simulink model "Motor_Load"  (R2025b)
settings: Solver=VariableStepAuto  StartTime=0.0  StopTime=400  MaxStep=0.002  RelTol=1e-3
model workspace (MAT data in the model file):
  CS_area_of_vehicle = 0.871
  Drag_coefficient = 0.195
  acceleration = 2.5
  air_density = 1.225
  gear_ratio = 5
  gravity = 9.81
  rolling_resistance = 0.05
  vehicle_mass = 180
  wheel_radius = 0.25
undefined symbols (not defined in the file or in its folder): Gradient_data, PMSM_Graph
settings Model: Creator=User  LastModifiedBy=User

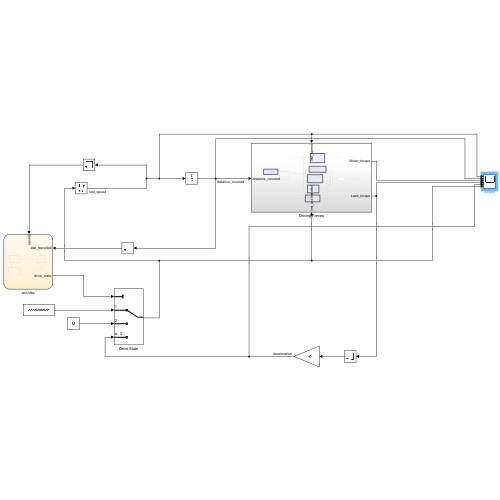
[thumbnail: Simulink's stored preview of the top-level diagram]
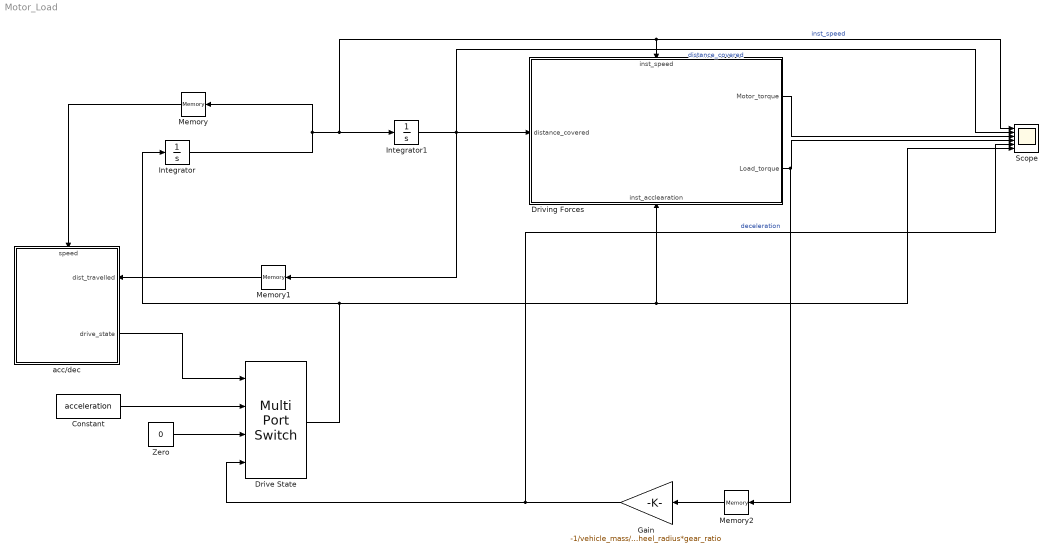
== system Motor_Load ==
  Constant : Constant  Value=acceleration
  Drive State : MultiPortSwitch  DataPortOrder=Specify indices  SaturateOnIntegerOverflow=off  InputSameDT=off
  Driving Forces : Subsystem
      settings: PortSchema="{\"entries\":[{\"content\":{\"sides\":[{\"content\":{\"connectorIds\":[\"In1\"]},\"type\":\"ConnectorPlacement.EquallySpacedRectSide\",\"uuid\":\"0ef3818d-e5de-4410-93cb-475bf6d7adfa\"},{\"content\":{\"connectorIds\":[\"Out1\",\"Out2\"],\"side\":\"RIGHT\"},\"type\":\"ConnectorPlacement.EquallySpacedRectSide\",\"uuid\":\"9d154a41-18f4-4f0c-ab8b-f09b7ff3397b\"},{\"content\":{\"connectorIds\":[\"In2\"],\"side\":\"TOP\"},\"type\":\"ConnectorPlacement.EquallySpacedRectSide\",\"uuid\":\"d46c2e69-b7e7-4a8c-bdbb-3c3b035d244f\"},{\"content\":{\"connectorIds\":[\"In3\"],\"side\":\"BOTTOM\"},\"type\":\"ConnectorPlacement.EquallySpacedRectSide\",\"uuid\":\"b2e27950-85a1-4e60-a0a3-1e85ddf78ec7\"}]},\"type\":\"ConnectorPlacement.EquallySpacedConnector\",\"uuid\":\"c1717862-f1cf-4e53-be39-73b9e4c32012\"}],\"packageUris\":[\"http://schema.mathworks.com/mf0/Connector/R2020b\"],\"version\":\"1.0\"}"
  Gain : Gain  Gain=-1/vehicle_mass/wheel_radius*gear_ratio
  Integrator : Integrator  InitialCondition=0.001  LimitOutput=on  UpperSaturationLimit=10  LowerSaturationLimit=-0.001
  Integrator1 : Integrator
  Memory : Memory
  Memory1 : Memory
  Memory2 : Memory
  Scope : Scope  NumInputPorts=6
      settings: ActiveDisplayYMinimum=-26.829853892938957  ActiveDisplayYMaximum=39.839891777673373
  Zero : Constant  Value=0  OutDataTypeStr=Inherit: Inherit via back propagation
  acc/dec : Stateflow chart  TreatAsAtomicUnit=on
      settings: PortSchema="{\"entries\":[{\"content\":{\"sides\":[{\"content\":{},\"type\":\"ConnectorPlacement.EquallySpacedRectSide\",\"uuid\":\"4b427815-5634-4ea7-8cfa-82438ecc852b\"},{\"content\":{\"connectorIds\":[\"In1\",\"Out1\"],\"side\":\"RIGHT\"},\"type\":\"ConnectorPlacement.EquallySpacedRectSide\",\"uuid\":\"a8ca7e8d-f0e3-4217-abff-5b21a522cee7\"},{\"content\":{\"connectorIds\":[\"In2\"],\"side\":\"TOP\"},\"type\":\"ConnectorPlacement.EquallySpacedRectSide\",\"uuid\":\"3ab37e47-b840-4f90-8038-0626af8ff66b\"}]},\"type\":\"ConnectorPlacement.EquallySpacedConnector\",\"uuid\":\"434126e8-21ff-4afc-bfcf-7bdbff78af77\"}],\"packageUris\":[\"http://schema.mathworks.com/mf0/Connector/R2020b\"],\"version\":\"1.0\"}"
  wires:
  Integrator/1 -> Memory/1, Integrator1/1, Scope/1, Driving Forces/2(inst_speed)  "inst_speed"
  Integrator1/1 -> Scope/2, Memory1/1, Driving Forces/1(distance_covered)  "distance_covered"
  Constant/1 -> Drive State/2
  acc/dec/1(drive_state) -> Drive State/1
  Gain/1 -> Scope/5, Drive State/4  "deceleration"
  Drive State/1 -> Driving Forces/3(inst_acclearation), Scope/6, Integrator/1
  Driving Forces/2(Load_torque) -> Memory2/1, Scope/4
  Driving Forces/1(Motor_torque) -> Scope/3
  Memory/1 -> acc/dec/2(speed)
  Zero/1 -> Drive State/3
  Memory1/1 -> acc/dec/1(dist_travelled)
  Memory2/1 -> Gain/1

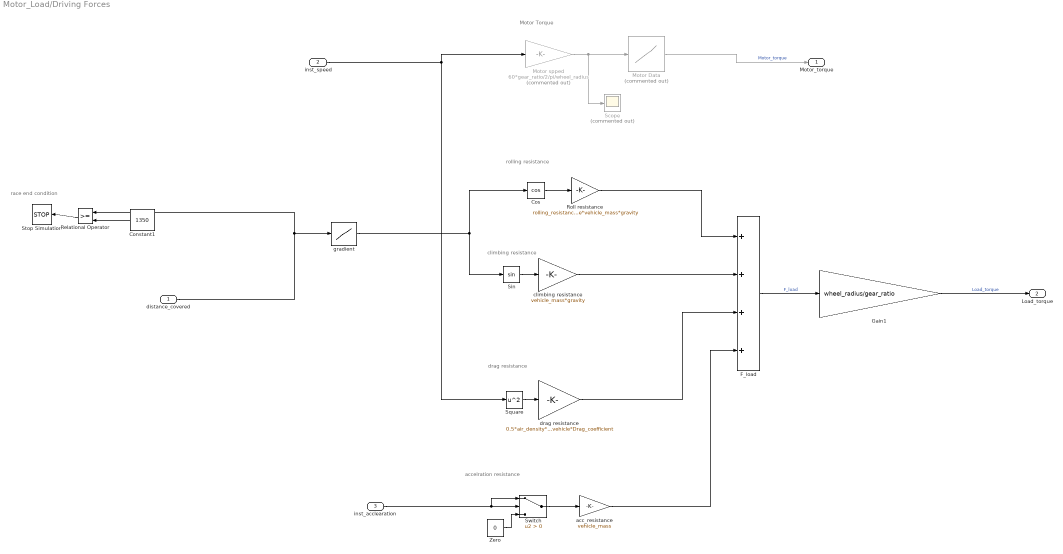
== system Motor_Load/Driving Forces ==
  note: Motor Torque
  note: race end condition
  note: climbing resistance
  note: rolling resistance
  note: drag resistance
  note: accelration resistance
  distance_covered : Inport
  inst_speed : Inport  Port=2
  inst_acclearation : Inport  Port=3
  Constant1 : Constant  Value=1350
  Cos : Trigonometry  Operator=cos
  F_load : Sum  Inputs=++++
  Gain1 : Gain  Gain=wheel_radius/gear_ratio
  Motor Data : Lookup_n-D  Commented=on  NumberOfTableDimensions=1  BreakpointsForDimension1=PMSM_Graph.Speed_RPM_  Table=PMSM_Graph.Torque_Nm_  InternalRulePriority=Speed  RndMeth=Simplest
  Motor spped : Gain  Commented=on  Gain=60*gear_ratio/2/pi/wheel_radius
  Relational Operator : RelationalOperator  OutDataTypeStr=boolean  RndMeth=Simplest
  Roll resistance : Gain  Gain=rolling_resistance*vehicle_mass*gravity
  Scope : Scope  Commented=on
      settings: ActiveDisplayYMinimum=-238.51755546466887  ActiveDisplayYMaximum=2148.5678584991233
  Sin : Trigonometry
  Square : Math  Operator=square
  Stop Simulation : Stop
  Switch : Switch  Criteria=u2 > Threshold  SaturateOnIntegerOverflow=off  InputSameDT=off
  Zero : Constant  Value=0  OutDataTypeStr=Inherit: Inherit via back propagation
  acc_resistance : Gain  Gain=vehicle_mass
  climbing resistance : Gain  Gain=vehicle_mass*gravity
  drag resistance : Gain  Gain=0.5*air_density*CS_area_of_vehicle*Drag_coefficient
  gradient : Lookup_n-D  NumberOfTableDimensions=1  BreakpointsForDimension1=Gradient_data.Distance  Table=Gradient_data.gradient  UseLastTableValue=on  InternalRulePriority=Speed  RndMeth=Simplest
  Motor_torque : Outport
  Load_torque : Outport  Port=2
  wires:
  Constant1/1 -> Relational Operator/2
  gradient/1 -> Sin/1, Cos/1
  Relational Operator/1 -> Stop Simulation/1
  Sin/1 -> climbing resistance/1
  distance_covered/1 -> Relational Operator/1, gradient/1
  Cos/1 -> Roll resistance/1
  drag resistance/1 -> F_load/3
  Square/1 -> drag resistance/1
  climbing resistance/1 -> F_load/2
  F_load/1 -> Gain1/1  "F_load"
  Gain1/1 -> Load_torque/1  "Load_torque"
  acc_resistance/1 -> F_load/4
  inst_acclearation/1 -> Switch/1, Switch/2
  Switch/1 -> acc_resistance/1
  Roll resistance/1 -> F_load/1
  inst_speed/1 -> Square/1, Motor spped/1
  Motor spped/1 -> Scope/1, Motor Data/1
  Motor Data/1 -> Motor_torque/1  "Motor_torque"
  Zero/1 -> Switch/3

== stateflow chart Motor_Load/acc//dec ==
  state Accleration
    entry: drive_state = 1;
  state Deceleration
    entry: drive_state = 3;
    exit: increment = 1;
  state Constant_speed
    entry: drive_state = 2;
  (default) -> Accleration
  Deceleration -> Accleration : [speed < 0]
  Accleration -> Constant_speed : [speed == 10]
  Constant_speed -> Deceleration : [dist_travelled > 1000 && increment == 0]
  data: dist_travelled input; speed input; increment local =0; drive_state output
